simulink model "power_dcdrive"  (Simulink 6.0)
settings: Solver=ode15s  SolverMode=SingleTasking  StartTime=0.0  StopTime=2.5
InitFcn:
  | load power_dcdrive_init
libraries: powerlib x11, simulink x2
Description:
  | The 'Model  initialization function' defined in the
  | 
  | Model Properties loads the  initial states vector
  | 
  | 'xInitial' saved in the power_dcdrive_init.mat file.
  | 
  | 
  | 
  | To start in steady state with Speed = 120 rad/s
  | 
  | and Torque = 5 N.m/s, check 'Initial state' in
  | 
  | Simulation/Simulation parameters/Workspace I/O.
settings Model: Creator=Hoand Lehuy, Laval University  LastModifiedBy=batserve  ExtModeTrigMode=oneshot  ExtModeArmWhenConnect=off  ExtModeAutoUpdateStatusClock=off
settings DataIOCC: LimitDataPoints=off  SaveFinalState=on  SaveOutput=off  SaveTime=off  SignalLoggingName=sigsOut
settings OptimizationCC: BlockReduction=off  BooleanDataType=off
settings DebuggingCC: CheckExecutionContextPreStartOutputMsg=on  CheckExecutionContextRuntimeOutputMsg=on  SolverPrmCheckMsg=none  UnconnectedInputMsg=none  UnconnectedOutputMsg=none
settings HardwareCC: TargetUnknown=on
settings RTWCC: TemplateMakefile=grt_unix.tmf

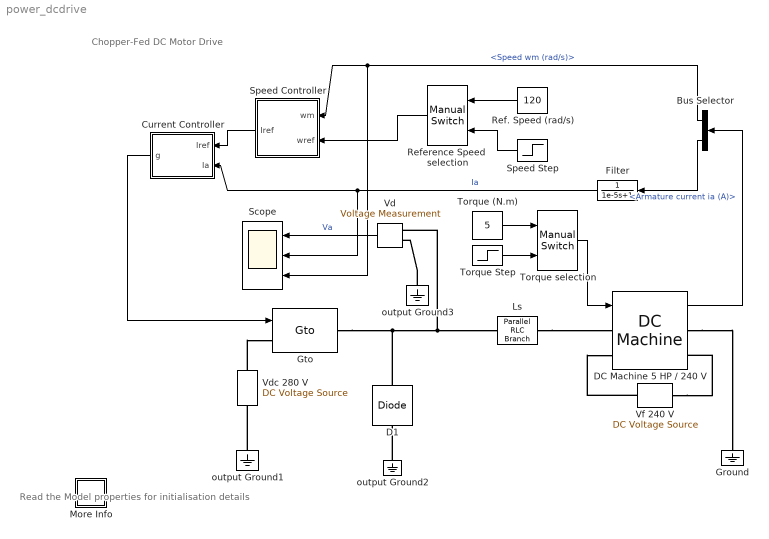
== system power_dcdrive ==
  note: Chopper-Fed DC Motor Drive
  note: Read the Model properties
      | for initialisation details
  Bus Selector : BusSelector  Orientation=left  DialogController=Simulink.DDGSource_Bus  OutputSignals=Speed wm (rad/s),Armature current ia (A)
  Current Controller : Subsystem  Orientation=left  mask{h=2}
      mask prompts: h "Hysteresis band (A)"
      mask help: Hysteresis Current Controller
      mask Display: plot(0,0,100,100,[45,45],[35,65],[55,55],[35,65],[45,65],[65,65],[35,55],[35,35])
  D1 : powerlib/Power Electronics/Diode  Orientation=up  Ron=0.05  Lon=5e-6  Vf=0.7  IC=0  Rs=Inf  Cs=0.1e-6  Measurements=off
  DC Machine 5 HP / 240 V : powerlib/Machines/DC Machine  PresetModel=No  ShowDetailedParameters=on  RLa="[ 0.5  0.01]"  RLf="[ 240  120]"  Laf=1.23  J=0.05  Bm=0.02  Tf=0  w0=0.1
  Filter : TransferFcn  Orientation=left  Numerator=1  Denominator=[1e-5 1]
      mask Display: disp('Filter')
  Ground : powerlib/Elements/Ground  Orientation=down  PhysicalDomain=powersysdomain  SubClassName=unknown  LeftPortType=p1  RightPortType=p1  LConnTagsString=a
  Gto : powerlib/Power Electronics/Gto  Ron=0.05  Lon=1e-6  Vf=1  Tf=1e-6  Tt=1e-6  IC=0  Rs=100  Cs=0.1e-6  Measurements=off
      settings: AttributesFormatString=\n
  Ls : powerlib/Elements/Parallel RLC Branch  PhysicalDomain=powersysdomain  SubClassName=unknown  LeftPortType=p1  RightPortType=p1  LConnTagsString=a  RConnTagsString=__new0  Resistance=inf  Inductance=10e-03  Capacitance=0  Measurements=None
  More Info : Subsystem
      mask Display: disp('?')
  Ref. Speed (rad/s) : Constant  Orientation=left  Value=120
  Reference Speed  selection : simulink/Signal Routing/Manual Switch  Orientation=left  sw=1  action=0
  Scope : Scope  NumInputPorts=3
      settings: TickLabels=on  YMin=-300~4.5~119.99  YMax=300~7.5~120.03  SaveName=var  Decimation=20
  Speed Controller : Subsystem  Orientation=left  mask(PI controller){Kp=1.6, Ki=16, Ilim=30}
      mask prompts: Kp "Proportional gain (Kp)"; Ki "Integral gain (Ki)"; Ilim "Current limit (A)"
      mask help: Proportional-Integral Speed Controller
      mask Display: plot(0,0,100,100,[35,35,65],[70,30,30],[35,65],[45,60])
  Speed Step : Step  Orientation=left  Time=0.4  Before=120  After=160  SampleTime=0
  Torque selection : simulink/Signal Routing/Manual Switch  sw=1  action=0
  Torque (N.m) : Constant  Value=5
  Torque Step : Step  Time=1.2  Before=5  After=25  SampleTime=0
  Vd : powerlib/Measurements/Voltage Measurement  Tag=PoWeRsYsTeMmEaSuReMeNt  Orientation=left  PhasorSimulation=off  OutputType=Magnitude  PSBequivalent=0
  "Vdc 280 V " : powerlib/Electrical Sources/DC Voltage Source  Description=source block  Orientation=up  Amplitude=280  Measurements=None
      settings: AttributesFormatString=\n
  Vf 240 V : powerlib/Electrical Sources/DC Voltage Source  Description=source block  Orientation=left  Amplitude=240  Measurements=None
      settings: AttributesFormatString=\n
  output Ground1 : powerlib/Elements/Ground  Orientation=down  PhysicalDomain=powersysdomain  SubClassName=unknown  LeftPortType=p1  RightPortType=p1  LConnTagsString=a
  output Ground2 : powerlib/Elements/Ground  Orientation=down  PhysicalDomain=powersysdomain  SubClassName=unknown  LeftPortType=p1  RightPortType=p1  LConnTagsString=a
  output Ground3 : powerlib/Elements/Ground  Orientation=down  PhysicalDomain=powersysdomain  SubClassName=unknown  LeftPortType=p1  RightPortType=p1  LConnTagsString=a
  wires:
  Speed Controller/1(Iref) -> Current Controller/1(Iref)
  Filter/1 -> Current Controller/2(Ia), Scope/2  "Ia"
  Bus Selector/1 -> Speed Controller/1(wm), Scope/3  "<Speed wm (rad/s)>"
  Bus Selector/2 -> Filter/1  "<Armature current ia (A)>"
  Current Controller/1(g) -> Gto/1
  Vd/1 -> Scope/1  "Va"
  DC Machine 5 HP / 240 V/1 -> Bus Selector/1
  Torque (N.m)/1 -> Torque selection/1
  Torque Step/1 -> Torque selection/2
  Torque selection/1 -> DC Machine 5 HP / 240 V/1
  Reference Speed  selection/1 -> Speed Controller/2(wref)
  Ref. Speed (rad/s)/1 -> Reference Speed  selection/1
  Speed Step/1 -> Reference Speed  selection/2
  connections:
  output Ground2/LConn1 -- D1/LConn1
  Gto/RConn1 -- Ls/LConn1 -- Vd/LConn1 -- D1/RConn1
  "Vdc 280 V "/RConn1 -- Gto/LConn1
  output Ground1/LConn1 -- "Vdc 280 V "/LConn1
  Ls/RConn1 -- DC Machine 5 HP / 240 V/LConn1
  output Ground3/LConn1 -- Vd/LConn2
  DC Machine 5 HP / 240 V/RConn1 -- Ground/LConn1
  Vf 240 V/LConn1 -- DC Machine 5 HP / 240 V/RConn2
  Vf 240 V/RConn1 -- DC Machine 5 HP / 240 V/LConn2

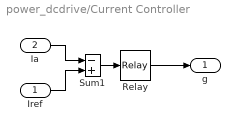
== system power_dcdrive/Current Controller ==
  Iref : Inport  Port=1  LatchInput=off
  Ia : Inport  Port=2  LatchInput=off
  Relay : Relay  OnSwitchValue=h/2  OffSwitchValue=-h/2
  Sum1 : Sum  Inputs=-+  SaturateOnIntegerOverflow=on  InputSameDT=on
  g : Outport  InitialOutput=0
  wires:
  Sum1/1 -> Relay/1
  Relay/1 -> g/1
  Ia/1 -> Sum1/1
  Iref/1 -> Sum1/2

== system power_dcdrive/More Info ==
  note: Start the simulation. Observe the motor current, voltage, and speed during the starting on the scope.
      |
      | At the end of the simulation time (1.5 s), the system has reached its steady-state. The final state vector can
      | be saved by previously  selecting 'Workspace I/O/Save to workspace/Final state' in Simulation/Parameters window.
      | Once the simultion is finished save the xFinal variable into xInitial.
      |
      | Note : The initial conditions state vector 'xInitial' to start with wm = 120 rad/s and TL = 5 N.m is stored in the
      |            'power_dcdrive_init.mat'  file. This vector is automatically loaded in your  workspace.
      |
      | Double click the two Manual Switch blocks to switch from  the constant wref and TL blocks to the Step blocks.
      | (Refence speed wref changed from 120 to 160 rad/s at t = 0.4 s and load torque changed from 5 to 25 N.m at  t= 1.2s).
      | In the Simulation/Simulation parameters/Workspace I/O menu check 'Initial state'  to use the xInitial vector of initial conditions.
      | Restart the simulation  and observe the drive response to successive changes in speed reference and load torque.
  note: Case study: Chopper-Fed DC Motor Drive
  note: Circuit Description
  note: Demonstration
  note: The DC motor is fed by the DC source through a chopper which consists of GTO thyristor Th1
      | and free-wheeling diode D1. The motor drives a mechanical load characterized by inertia J, friction
      | coeficient B, and load torque TL.
      |
      | The hysteresis current controller compares the sensed current with the reference and generates
      | the trigger signal for the GTO thyristor to force the motor current to follow the reference.
      | The speed control loop uses a proportional-integral controller which produces the reference for the current loop.
      | Current and Voltage Measurement blocks provide signals for visualization purpose.
  note: H. Le-Huy (Universite Laval, Quebec)

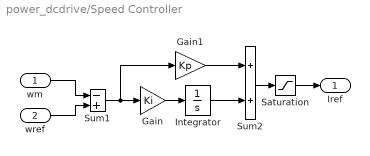
== system power_dcdrive/Speed Controller ==
  wm : Inport  Port=1  LatchInput=off
  wref : Inport  Port=2  LatchInput=off
  Gain : Gain  Gain=Ki  SaturateOnIntegerOverflow=on
  Gain1 : Gain  Gain=Kp  SaturateOnIntegerOverflow=on
  Integrator : Integrator  LimitOutput=on  UpperSaturationLimit=Ilim  LowerSaturationLimit=-Ilim
  Saturation : Saturate  UpperLimit=Ilim  LowerLimit=-Ilim
  Sum1 : Sum  Inputs=-+  SaturateOnIntegerOverflow=on  InputSameDT=on
  Sum2 : Sum  SaturateOnIntegerOverflow=on  InputSameDT=on
  Iref : Outport  InitialOutput=0
  wires:
  Saturation/1 -> Iref/1
  Sum2/1 -> Saturation/1
  Integrator/1 -> Sum2/2
  wref/1 -> Sum1/2
  wm/1 -> Sum1/1
  Sum1/1 -> Gain1/1, Gain/1
  Gain/1 -> Integrator/1
  Gain1/1 -> Sum2/1
